simulink model "QAM"  (R2018b)
settings: Solver=VariableStepAuto  StartTime=0.0  StopTime=0.1  FixedStep=10e-6  RelTol=10e-3
libraries: dspsrcs4 x4, commrandsrc3 x3, commdigbbndpm3 x1, commdigbbndam3 x1
settings Model: Creator=marcone  LastModifiedBy=marcone

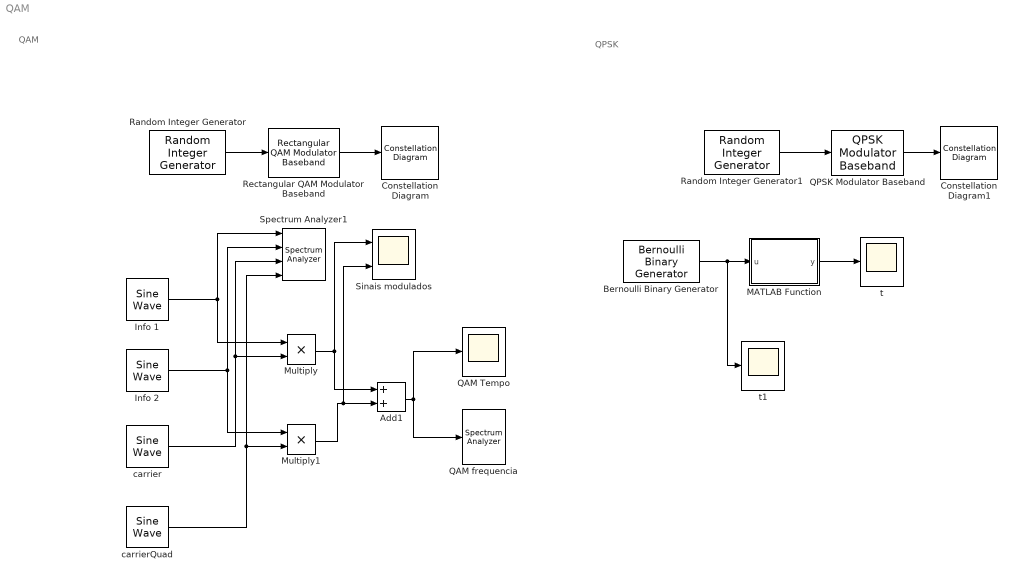
== system QAM ==
  note: QPSK
  note: QAM
  Add1 : Sum
  Bernoulli Binary Generator : commrandsrc3/Bernoulli Binary Generator  ProbabilityOfZero=0.5  SeedSource=Auto  Seed=0  SampleTime=1  SamplesPerFrame=1  OutputDataType=double  SimulateUsing=Interpreted execution
  Constellation Diagram : ConstellationDiagram
  Constellation Diagram1 : ConstellationDiagram
  Info 1 : dspsrcs4/Sine Wave  Amplitude=0.3  Frequency=2e3  Phase=0  SampleMode=Discrete  OutComplex=Real  CompMethod=Trigonometric fcn  TableSize=Speed  SampleTime=1/1e6  SamplesPerFrame=100  ResetState=Restart at time zero  OutputFrames=off  dataType=double  wordLen=16  udDataType=sfix(16)  fracBitsMode=Best precision  numFracBits=15  OutDataTypeStr=double  LastOutDataTypeStr=double
  Info 2 : dspsrcs4/Sine Wave  Amplitude=0.5  Frequency=7e3  Phase=0  SampleMode=Discrete  OutComplex=Real  CompMethod=Trigonometric fcn  TableSize=Speed  SampleTime=1/1e6  SamplesPerFrame=100  ResetState=Restart at time zero  OutputFrames=off  dataType=double  wordLen=16  udDataType=sfix(16)  fracBitsMode=Best precision  numFracBits=15  OutDataTypeStr=double  LastOutDataTypeStr=double
  MATLAB Function : MATLAB Function  TreatAsAtomicUnit=on
  Multiply : Product
  Multiply1 : Product
  QAM Tempo : Scope
  QAM frequencia : SpectrumAnalyzer
  QPSK Modulator Baseband : commdigbbndpm3/QPSK Modulator Baseband  InType=Integer  Enc=Gray  Ph=pi/4  outDtype=double  outWordLen=16  outUDDataType=sfix(16)  outFracLenMode=Best precision  outFracLen=15  outDataTypeStr=double  outLastDataTypeStr=double
  Random Integer Generator : commrandsrc3/Random Integer Generator  SetSize=4  SeedSource=Auto  Seed=0  SampleTime=1  SamplesPerFrame=10000  OutputDataType=double  SimulateUsing=Interpreted execution
  Random Integer Generator1 : commrandsrc3/Random Integer Generator  SetSize=4  SeedSource=Auto  Seed=0  SampleTime=1  SamplesPerFrame=10000  OutputDataType=double  SimulateUsing=Interpreted execution
  Rectangular QAM Modulator Baseband : commdigbbndam3/Rectangular QAM Modulator Baseband  M=4  InType=Integer  Enc=Gray  Mapping=[0:15]  PowType=Min. distance between symbols  MinDist=2  AvgPow=1  PeakPow=1  Ph=0  outDtype=double  outWordLen=16  outUDDataType=sfix(16)  outFracLenMode=Best precision  outFracLen=15  outDataTypeStr=double  outLastDataTypeStr=double
  Sinais modulados : Scope  NumInputPorts=2
  Spectrum Analyzer1 : SpectrumAnalyzer  NumInputPorts=4
  carrier : dspsrcs4/Sine Wave  Amplitude=2  Frequency=100e3  Phase=0  SampleMode=Discrete  OutComplex=Real  CompMethod=Trigonometric fcn  TableSize=Speed  SampleTime=1/1e6  SamplesPerFrame=100  ResetState=Restart at time zero  OutputFrames=off  dataType=double  wordLen=16  udDataType=sfix(16)  fracBitsMode=Best precision  numFracBits=15  OutDataTypeStr=double  LastOutDataTypeStr=double
  carrierQuad : dspsrcs4/Sine Wave  Amplitude=2  Frequency=100e3  Phase=90*pi/180  SampleMode=Discrete  OutComplex=Real  CompMethod=Trigonometric fcn  TableSize=Speed  SampleTime=1/1e6  SamplesPerFrame=100  ResetState=Restart at time zero  OutputFrames=off  dataType=double  wordLen=16  udDataType=sfix(16)  fracBitsMode=Best precision  numFracBits=15  OutDataTypeStr=double  LastOutDataTypeStr=double
  t : Scope
  t1 : Scope
  wires:
  Info 1/1 -> Multiply/1, Spectrum Analyzer1/1
  Info 2/1 -> Multiply1/1, Spectrum Analyzer1/2
  carrier/1 -> Multiply/2, Spectrum Analyzer1/3
  carrierQuad/1 -> Spectrum Analyzer1/4, Multiply1/2
  Multiply/1 -> Add1/1, Sinais modulados/1
  Multiply1/1 -> Sinais modulados/2, Add1/2
  Add1/1 -> QAM Tempo/1, QAM frequencia/1
  Random Integer Generator/1 -> Rectangular QAM Modulator Baseband/1
  Rectangular QAM Modulator Baseband/1 -> Constellation Diagram/1
  Random Integer Generator1/1 -> QPSK Modulator Baseband/1
  QPSK Modulator Baseband/1 -> Constellation Diagram1/1
  Bernoulli Binary Generator/1 -> t1/1, MATLAB Function/1(u)
  MATLAB Function/1(y) -> t/1

== matlab function QAM/MATLAB Function ==
  data: u input; y output
function y = fcn(u)

if u == 1
    y = 1;
else
    y = -1;
end
